simulink model "block model"  (R2020b)
settings: Solver=FixedStepAuto  StartTime=0.0  StopTime=10.0  RelTol=1e-3  EnableMultiTasking=on
libraries: arduinolib x5, realtime_examples_misc x1
settings Model: SimulationMode=external  SILPILModeSetting=veronly  ExtModeTrigDuration=2  Creator=Castoleru  LastModifiedBy=Castoleru
settings OptimizationCC: EnhancedBackFolding=on  PassReuseOutputArgsAs=Individual arguments  ZeroExternalMemoryAtStartup=off  ZeroInternalMemoryAtStartup=off  MaxStackSize=64  OptimizeBlockOrder=speed  DifferentSizesBufferReuse=on  OptimizationCustomize=off  EfficientTunableParamExpr=on
settings DebuggingCC: ParameterTunabilityLossMsg=error
settings HardwareCC: ProdBitPerInt=16  ProdBitPerPointer=16  ProdBitPerSizeT=16  ProdBitPerPtrDiffT=16  ProdLargestAtomicFloat=None  ProdWordSize=8  ProdHWDeviceType=Atmel->AVR
settings SFSimCC: MATLABDynamicMemAlloc=off
settings RTWCC: Description=Embedded Coder  SystemTargetFile=ert.tlc  HardwareBoard=Arduino Uno  TemplateMakefile=ert_default_tmf  Toolchain=Arduino AVR  BuildConfiguration=Faster Runs
settings CodeAppCC: ForceParamTrailComments=on  IgnoreCustomStorageClasses=off  OperatorAnnotations=on  SimulinkDataObjDesc=on  SFDataObjDesc=on  InsertBlockDesc=on
settings ERTTargetCC: SupportContinuousTime=on  SupportVariableSizeSignals=on  ExtModeStaticAllocSize=250

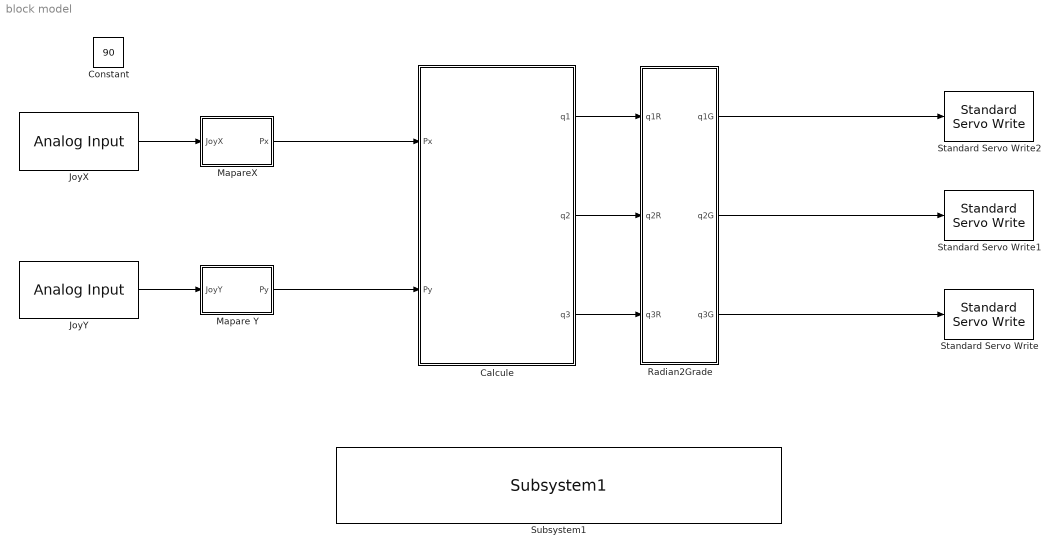
== system block model ==
  Calcule : MATLAB Function  TreatAsAtomicUnit=on
  Constant : Constant  Value=90
  JoyX : arduinolib/Analog Input  pinNumber=0  ReadResultsOnly=off  ConversionTriggerSource=Software  ExternalTriggerType=uint32( 0 )  OutputDataType=uint16  EnableConversionCompleteNotify=off  EnableOuputStatus=off  SampleTime=1  blockPlatform=arduino
  JoyY : arduinolib/Analog Input  pinNumber=1  ReadResultsOnly=off  ConversionTriggerSource=Software  ExternalTriggerType=uint32( 0 )  OutputDataType=uint16  EnableConversionCompleteNotify=off  EnableOuputStatus=off  SampleTime=1  blockPlatform=arduino
  Mapare Y : MATLAB Function  TreatAsAtomicUnit=on
  MapareX : MATLAB Function  TreatAsAtomicUnit=on
  Radian2Grade : MATLAB Function  TreatAsAtomicUnit=on
  Standard Servo Write : arduinolib/Standard Servo Write  pinNumber=3  ServoIndex=0  blockPlatform=arduino
  Standard Servo Write1 : arduinolib/Standard Servo Write  pinNumber=10  ServoIndex=1  blockPlatform=arduino
  Standard Servo Write2 : arduinolib/Standard Servo Write  pinNumber=11  ServoIndex=2  blockPlatform=arduino
  Subsystem1 : realtime_examples_misc/Subsystem1  SystemSampleTime=-1  VariantActivationTime=update diagram  Latency=0  AutoFrameSizeCalculation=off
      settings: SourceProductBaseCode=SL
  wires:
  Calcule/3(q3) -> Radian2Grade/3(q3R)
  Radian2Grade/3(q3G) -> Standard Servo Write/1
  JoyY/1 -> Mapare Y/1(JoyY)
  Mapare Y/1(Py) -> Calcule/2(Py)
  Calcule/1(q1) -> Radian2Grade/1(q1R)
  Radian2Grade/1(q1G) -> Standard Servo Write2/1
  JoyX/1 -> MapareX/1(JoyX)
  MapareX/1(Px) -> Calcule/1(Px)
  Calcule/2(q2) -> Radian2Grade/2(q2R)
  Radian2Grade/2(q2G) -> Standard Servo Write1/1

== matlab function block model/Mapare Y ==
  data: JoyY input; Py output
function Py = fcn(JoyY)
   JoyY = double(JoyY);
   if JoyY  > 512
       JoyY = 512;
   end
   Py = ((8/512) * JoyY);
end

== matlab function block model/MapareX ==
  data: JoyX input; Px output
function Px = fcn(JoyX)
    JoyX = double(JoyX);
    Px = ((16/1023) * JoyX) - 8;
end

== matlab function block model/Calcule ==
  data: Px input; q1 output; Py input; q2 output; q3 output
function [q1,q2,q3] = fcn(Px,Py)
    Px = double(Px);
    Py = double(Py);
    Pz = 14;
    q1 = -atan(Px/Py);
    q2 = -2*atan((-(132*cos(q1)^2 + Pz^2*cos(q1)^2 + Py^2 - 28*Pz*cos(q1)^2)*...
    (180*cos(q1)^2 + Pz^2*cos(q1)^2 + Py^2 - 28*Pz*cos(q1)^2))^(1/2)/...
    (180*cos(q1)^2 + Pz^2*cos(q1)^2 + Py^2 - 28*Pz*cos(q1)^2));
    q3 = 2*atan((-(132*cos(q1)^2 + Pz^2*cos(q1)^2 + Py^2 - 28*Pz*cos(q1)^2)* ...
    (180*cos(q1)^2 + Pz^2*cos(q1)^2 + Py^2 - 28*Pz*cos(q1)^2))^(1/2)/...
    (180*cos(q1)^2 + Pz^2*cos(q1)^2 + Py^2 - 28*Pz*cos(q1)^2));
    
end

== matlab function block model/Radian2Grade ==
  data: q1R input; q1G output; q2R input; q3R input; q2G output; q3G output
function [q1G,q2G,q3G] = fcn(q1R,q2R,q3R)

    q1G = (q1R*180/pi) +90;
    q2G = ((q2R*180/pi))/2;    
    q3G = ((q3R*180/pi))/2;
end
